simulink library "lib_rfsoc_fec"  (R2020b)
settings: Solver=VariableStepAuto  StartTime=0.0  StopTime=10.0  RelTol=1e-3
undefined symbols (not defined in the file): d, fs
libraries: hdlsllib x42, commseqgen3 x28, simulink x17, dspsigops x10
(part 1 of 2)
settings Model: Creator=ckb13136  LastModifiedBy=ckb13136

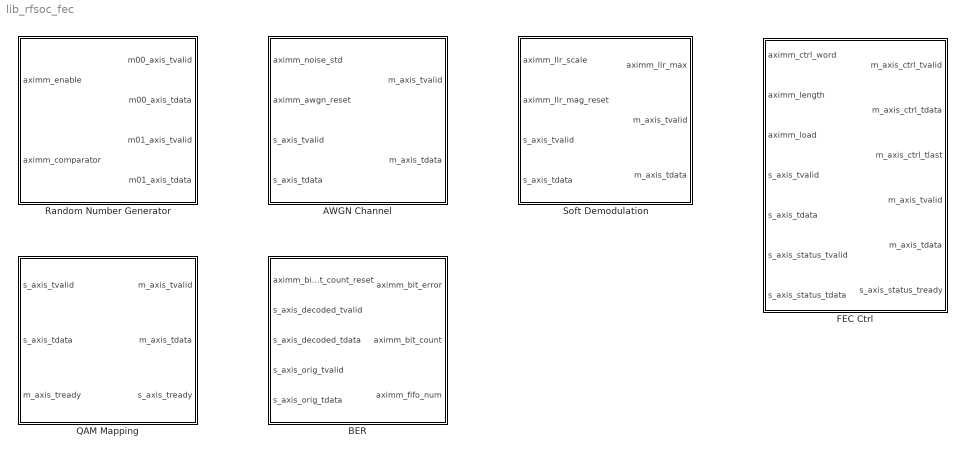
== system lib_rfsoc_fec ==
  AWGN Channel : Subsystem  TreatAsAtomicUnit=on
  BER : Subsystem  TreatAsAtomicUnit=on
  FEC Ctrl : Subsystem  TreatAsAtomicUnit=on
  QAM Mapping : Subsystem  TreatAsAtomicUnit=on
  Random Number Generator : Subsystem  TreatAsAtomicUnit=on
  Soft Demodulation : Subsystem  TreatAsAtomicUnit=on

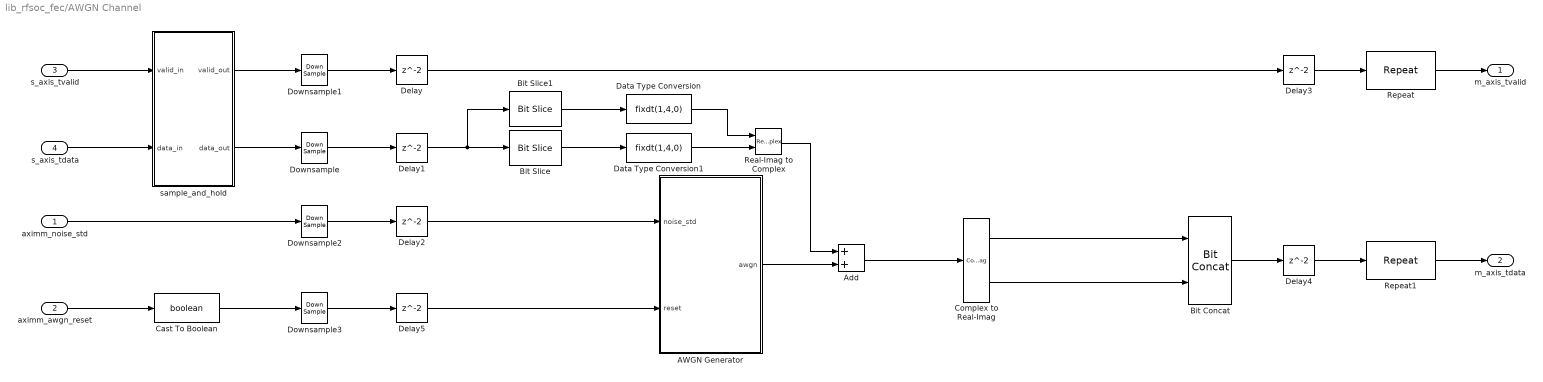
== system lib_rfsoc_fec/AWGN Channel ==
  aximm_noise_std : Inport
  aximm_awgn_reset : Inport  Port=2
  s_axis_tvalid : Inport  Port=3
  s_axis_tdata : Inport  Port=4
  AWGN Generator : Subsystem
  Add : Sum  OutDataTypeStr=fixdt(1,16,11)  SaturateOnIntegerOverflow=on
  Bit Concat : hdlsllib/Logic and Bit Operations/Bit Concat  numInputs=2
  Bit Slice : hdlsllib/Logic and Bit Operations/Bit Slice  lidx=3  ridx=0
      settings: SourceProductBaseCode=SL
  Bit Slice1 : hdlsllib/Logic and Bit Operations/Bit Slice  lidx=7  ridx=4
      settings: SourceProductBaseCode=SL
  Cast To Boolean : DataTypeConversion  OutDataTypeStr=boolean
  Complex to Real-Imag : ComplexToRealImag
  Data Type Conversion : DataTypeConversion  OutDataTypeStr=fixdt(1,4,0)  ConvertRealWorld=Stored Integer (SI)
  Data Type Conversion1 : DataTypeConversion  OutDataTypeStr=fixdt(1,4,0)  ConvertRealWorld=Stored Integer (SI)
  Delay{,1..5} (6 alike) : Delay
  Downsample{,1..3} (4 alike) : DownSample  N=4  RateOptions=Allow multirate processing
  Real-Imag to Complex : RealImagToComplex
  Repeat : dspsigops/Repeat  N=4  InputProcessing=Columns as channels (frame based)  RateOptions=Allow multirate processing  ic=0  mode=Unused parameter value
      settings: SourceProductName=DSP System Toolbox
  Repeat1 : dspsigops/Repeat  N=4  InputProcessing=Columns as channels (frame based)  RateOptions=Allow multirate processing  ic=0  mode=Unused parameter value
      settings: SourceProductName=DSP System Toolbox
  sample_and_hold : Subsystem
  m_axis_tvalid : Outport
  m_axis_tdata : Outport  Port=2
  wires:
  AWGN Generator/1(awgn) -> Add/2
  aximm_noise_std/1 -> Downsample2/1
  Delay2/1 -> AWGN Generator/1(noise_std)
  Downsample2/1 -> Delay2/1
  Delay5/1 -> AWGN Generator/2(reset)
  sample_and_hold/1(" valid_out") -> Downsample1/1
  Downsample1/1 -> Delay/1
  Downsample/1 -> Delay1/1
  Delay/1 -> Delay3/1
  sample_and_hold/2(" data_out") -> Downsample/1
  s_axis_tvalid/1 -> sample_and_hold/1(valid_in)
  s_axis_tdata/1 -> sample_and_hold/2(data_in)
  Delay1/1 -> Bit Slice1/1, Bit Slice/1
  Repeat1/1 -> m_axis_tdata/1
  Repeat/1 -> m_axis_tvalid/1
  Delay3/1 -> Repeat/1
  Delay4/1 -> Repeat1/1
  Bit Slice1/1 -> Data Type Conversion/1
  Bit Slice/1 -> Data Type Conversion1/1
  Data Type Conversion/1 -> Real-Imag to Complex/1
  Data Type Conversion1/1 -> Real-Imag to Complex/2
  Real-Imag to Complex/1 -> Add/1
  Add/1 -> Complex to Real-Imag/1
  Bit Concat/1 -> Delay4/1
  Complex to Real-Imag/1 -> Bit Concat/1
  Complex to Real-Imag/2 -> Bit Concat/2
  Downsample3/1 -> Delay5/1
  aximm_awgn_reset/1 -> Cast To Boolean/1
  Cast To Boolean/1 -> Downsample3/1

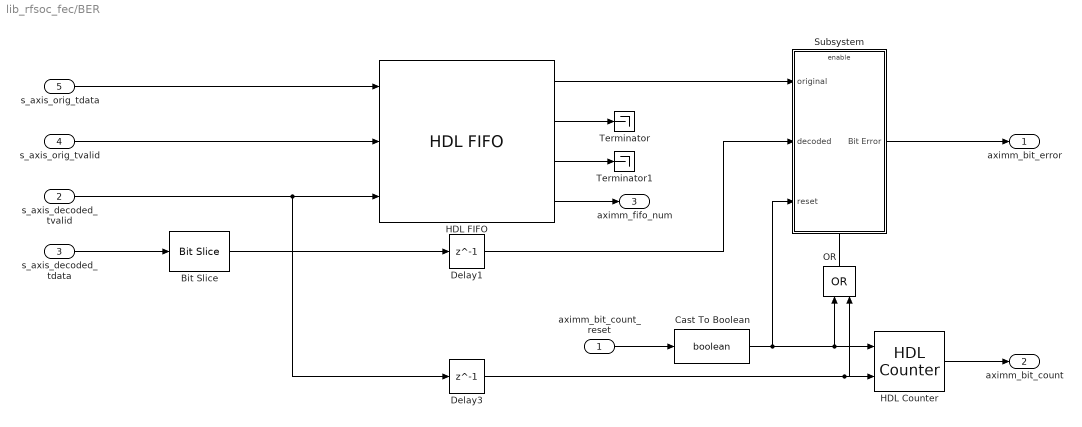
== system lib_rfsoc_fec/BER ==
  aximm_bit_count_reset : Inport
  s_axis_decoded_tvalid : Inport  Port=2
  s_axis_decoded_tdata : Inport  Port=3
  s_axis_orig_tvalid : Inport  Port=4
  s_axis_orig_tdata : Inport  Port=5
  Bit Slice : hdlsllib/Logic and Bit Operations/Bit Slice  lidx=7  ridx=0
      settings: SourceProductBaseCode=SL
  Cast To Boolean : DataTypeConversion  OutDataTypeStr=boolean
  Delay1 : Delay  DelayLength=1
  Delay3 : Delay  DelayLength=1
  HDL Counter : hdlsllib/Sources/HDL Counter  CountType=Free running  CountInit=0  CountStep=8  CountMax=25  CountFromType=Initial value  CountFrom=0  CountResetPort=on  CountLoadPort=off  CountEnbPort=on  CountDirPort=off  CountDataType=Unsigned  CountWordLen=32  CountFracLen=0  CountSampTime=1
  HDL FIFO : hdlsllib/HDL RAMs/HDL FIFO  fifo_size=8192  mode=Classic  ratio=1  push_msg=Warning  pop_msg=Warning  show_empty=on  show_full=on  show_num=on  LabelModeActiveChoice_Mode=Classic
      settings: SourceProductBaseCode=SL
  OR : Logic  Operator=OR  IconShape=distinctive  AllPortsSameDT=off  OutDataTypeStr=boolean
  Subsystem : Subsystem
  Terminator : Terminator
  Terminator1 : Terminator
  aximm_bit_error : Outport
  aximm_bit_count : Outport  Port=2
  aximm_fifo_num : Outport  Port=3
  wires:
  HDL FIFO/4 -> aximm_fifo_num/1
  HDL FIFO/2 -> Terminator/1
  s_axis_decoded_tvalid/1 -> HDL FIFO/3, Delay3/1
  Delay3/1 -> OR/2, HDL Counter/2
  s_axis_decoded_tdata/1 -> Bit Slice/1
  s_axis_orig_tvalid/1 -> HDL FIFO/2
  HDL FIFO/3 -> Terminator1/1
  Subsystem/1(Bit Error) -> aximm_bit_error/1
  HDL FIFO/1 -> Subsystem/1(original)
  Delay1/1 -> Subsystem/2(decoded)
  HDL Counter/1 -> aximm_bit_count/1
  Bit Slice/1 -> Delay1/1
  s_axis_orig_tdata/1 -> HDL FIFO/1
  aximm_bit_count_reset/1 -> Cast To Boolean/1
  Cast To Boolean/1 -> OR/1, HDL Counter/1, Subsystem/3(reset)
  OR/1 -> Subsystem/Enable

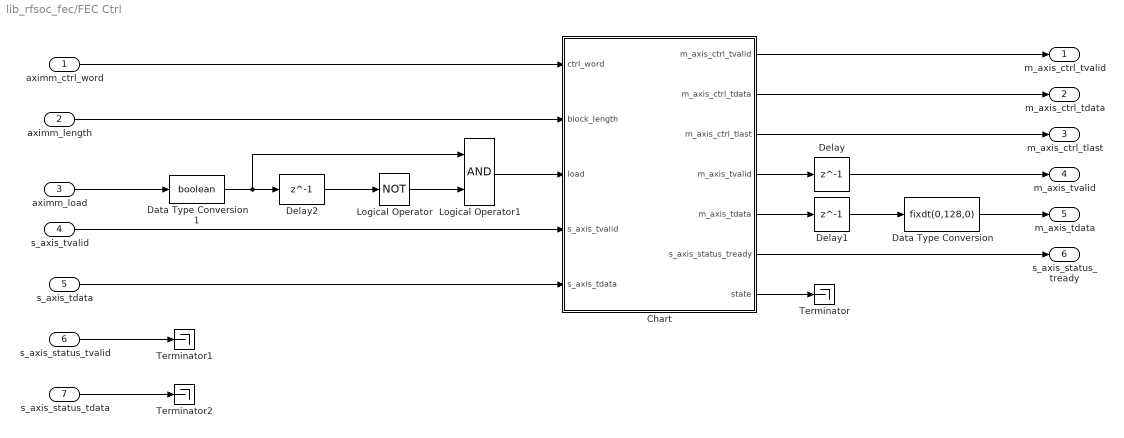
== system lib_rfsoc_fec/FEC Ctrl ==
  aximm_ctrl_word : Inport
  aximm_length : Inport  Port=2
  aximm_load : Inport  Port=3
  s_axis_tvalid : Inport  Port=4
  s_axis_tdata : Inport  Port=5
  s_axis_status_tvalid : Inport  Port=6
  s_axis_status_tdata : Inport  Port=7
  Chart : Stateflow chart  TreatAsAtomicUnit=on
  Data Type Conversion : DataTypeConversion  OutDataTypeStr=fixdt(0,128,0)
  Data Type Conversion1 : DataTypeConversion  OutDataTypeStr=boolean  SaturateOnIntegerOverflow=on  RndMeth=Zero
  Delay : Delay  DelayLength=1
  Delay1 : Delay  DelayLength=1
  Delay2 : Delay  DelayLength=1  InitialCondition=1  InputProcessing=Columns as channels (frame based)
  Logical Operator : Logic  Operator=NOT  Inputs=1
  Logical Operator1 : Logic
  Terminator : Terminator
  Terminator1 : Terminator
  Terminator2 : Terminator
  m_axis_ctrl_tvalid : Outport
  m_axis_ctrl_tdata : Outport  Port=2
  m_axis_ctrl_tlast : Outport  Port=3
  m_axis_tvalid : Outport  Port=4
  m_axis_tdata : Outport  Port=5
  s_axis_status_tready : Outport  Port=6
  wires:
  Chart/3(m_axis_ctrl_tlast) -> m_axis_ctrl_tlast/1
  Chart/7(state) -> Terminator/1
  aximm_length/1 -> Chart/2(block_length)
  s_axis_tvalid/1 -> Chart/4(s_axis_tvalid)
  s_axis_tdata/1 -> Chart/5(s_axis_tdata)
  aximm_ctrl_word/1 -> Chart/1(ctrl_word)
  Chart/2(m_axis_ctrl_tdata) -> m_axis_ctrl_tdata/1
  Chart/4(m_axis_tvalid) -> Delay/1
  Chart/5(m_axis_tdata) -> Delay1/1
  Chart/6(s_axis_status_tready) -> s_axis_status_tready/1
  Chart/1(m_axis_ctrl_tvalid) -> m_axis_ctrl_tvalid/1
  Delay/1 -> m_axis_tvalid/1
  Delay1/1 -> Data Type Conversion/1
  Data Type Conversion/1 -> m_axis_tdata/1
  Logical Operator1/1 -> Chart/3(load)
  s_axis_status_tvalid/1 -> Terminator1/1
  s_axis_status_tdata/1 -> Terminator2/1
  Logical Operator/1 -> Logical Operator1/2
  Data Type Conversion1/1 -> Delay2/1, Logical Operator1/1
  Delay2/1 -> Logical Operator/1
  aximm_load/1 -> Data Type Conversion1/1

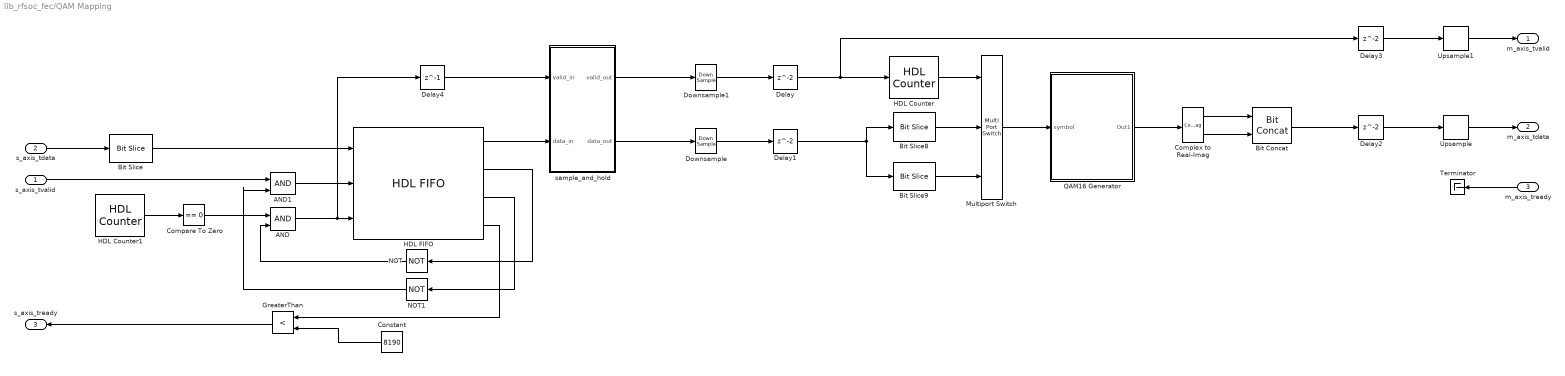
== system lib_rfsoc_fec/QAM Mapping ==
  s_axis_tvalid : Inport
  s_axis_tdata : Inport  Port=2
  m_axis_tready : Inport  Port=3
  AND : Logic  IconShape=distinctive  AllPortsSameDT=off  OutDataTypeStr=boolean
  AND1 : Logic  IconShape=distinctive  AllPortsSameDT=off  OutDataTypeStr=boolean
  Bit Concat : hdlsllib/Logic and Bit Operations/Bit Concat  numInputs=2
  Bit Slice : hdlsllib/Logic and Bit Operations/Bit Slice  lidx=7  ridx=0
      settings: SourceProductBaseCode=SL
  Bit Slice8 : hdlsllib/Logic and Bit Operations/Bit Slice  lidx=3  ridx=0
      settings: SourceProductBaseCode=SL
  Bit Slice9 : hdlsllib/Logic and Bit Operations/Bit Slice  lidx=7  ridx=4
      settings: SourceProductBaseCode=SL
  Compare To Zero : simulink/Logic and Bit Operations/Compare To Zero  relop===  OutDataTypeStr=boolean
  Complex to Real-Imag : ComplexToRealImag
  Constant : Constant  Value=8190  OutDataTypeStr=fixdt(0,log2(8190),0)  SampleTime=1/(fs*16)
  Delay{,1..3} (4 alike) : Delay
  Delay4 : Delay  DelayLength=1
  Downsample : DownSample  N=4  RateOptions=Allow multirate processing
  Downsample1 : DownSample  N=4  RateOptions=Allow multirate processing
  GreaterThan : RelationalOperator  Operator=<  OutDataTypeStr=boolean  RndMeth=Simplest
  HDL Counter : hdlsllib/Sources/HDL Counter  CountType=Count limited  CountInit=0  CountStep=1  CountMax=1  CountFromType=Initial value  CountFrom=0  CountResetPort=off  CountLoadPort=off  CountEnbPort=on  CountDirPort=off  CountDataType=Unsigned  CountWordLen=1  CountFracLen=0  CountSampTime=1/(fs*2)
  HDL Counter1 : hdlsllib/Sources/HDL Counter  CountType=Free running  CountInit=0  CountStep=1  CountMax=1  CountFromType=Initial value  CountFrom=0  CountResetPort=off  CountLoadPort=off  CountEnbPort=off  CountDirPort=off  CountDataType=Unsigned  CountWordLen=3  CountFracLen=0  CountSampTime=1/(fs*16)
  HDL FIFO : hdlsllib/HDL RAMs/HDL FIFO  fifo_size=8192  mode=Classic  ratio=1  push_msg=Warning  pop_msg=Warning  show_empty=on  show_full=on  show_num=on  LabelModeActiveChoice_Mode=Classic
      settings: SourceProductBaseCode=SL
  Multiport Switch : MultiPortSwitch  DataPortOrder=Zero-based contiguous  Inputs=2  zeroidx=on
  NOT : Logic  Operator=NOT  IconShape=distinctive  AllPortsSameDT=off  OutDataTypeStr=boolean
  NOT1 : Logic  Operator=NOT  IconShape=distinctive  AllPortsSameDT=off  OutDataTypeStr=boolean
  QAM16 Generator : Subsystem
  Terminator : Terminator
  Upsample : dspsigops/Upsample  N=4  phase=0  RateOptions=Allow multirate processing  ic=0  mode=Unused parameter value
  Upsample1 : dspsigops/Upsample  N=4  phase=0  RateOptions=Allow multirate processing  ic=0  mode=Unused parameter value
  sample_and_hold : Subsystem
  m_axis_tvalid : Outport
  m_axis_tdata : Outport  Port=2
  s_axis_tready : Outport  Port=3
  wires:
  Bit Slice9/1 -> Multiport Switch/3
  Bit Slice8/1 -> Multiport Switch/2
  HDL Counter/1 -> Multiport Switch/1
  Multiport Switch/1 -> QAM16 Generator/1(symbol)
  Downsample/1 -> Delay1/1
  sample_and_hold/1(" valid_out") -> Downsample1/1
  sample_and_hold/2(" data_out") -> Downsample/1
  Downsample1/1 -> Delay/1
  HDL FIFO/1 -> sample_and_hold/2(data_in)
  Delay/1 -> Delay3/1, HDL Counter/1
  Delay1/1 -> Bit Slice9/1, Bit Slice8/1
  Delay2/1 -> Upsample/1
  Delay3/1 -> Upsample1/1
  Upsample1/1 -> m_axis_tvalid/1
  Upsample/1 -> m_axis_tdata/1
  QAM16 Generator/1(Out1) -> Complex to Real-Imag/1
  Complex to Real-Imag/1 -> Bit Concat/1
  Complex to Real-Imag/2 -> Bit Concat/2
  Bit Concat/1 -> Delay2/1
  m_axis_tready/1 -> Terminator/1
  s_axis_tvalid/1 -> AND1/1
  s_axis_tdata/1 -> Bit Slice/1
  Bit Slice/1 -> HDL FIFO/1
  HDL FIFO/2 -> NOT/1
  AND/1 -> Delay4/1, HDL FIFO/3
  NOT/1 -> AND/2
  Constant/1 -> GreaterThan/2
  AND1/1 -> HDL FIFO/2
  HDL FIFO/3 -> NOT1/1
  NOT1/1 -> AND1/2
  HDL FIFO/4 -> GreaterThan/1
  GreaterThan/1 -> s_axis_tready/1
  HDL Counter1/1 -> Compare To Zero/1
  Compare To Zero/1 -> AND/1
  Delay4/1 -> sample_and_hold/1(valid_in)

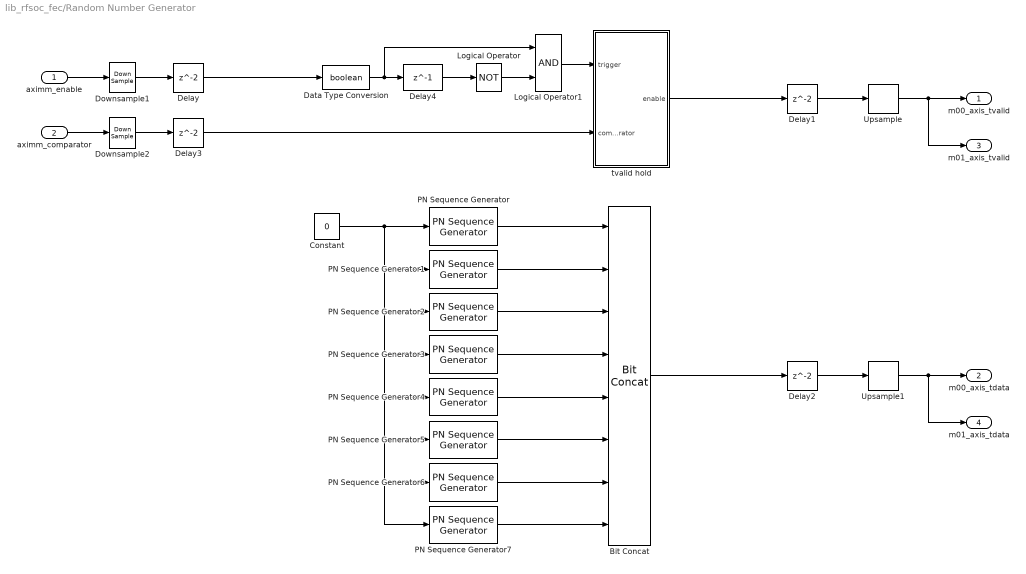
== system lib_rfsoc_fec/Random Number Generator ==
  aximm_enable : Inport
  aximm_comparator : Inport  Port=2
  Bit Concat : hdlsllib/Logic and Bit Operations/Bit Concat  numInputs=8
  Constant : Constant  Value=0  OutDataTypeStr=boolean  SampleTime=1/fs
  Data Type Conversion : DataTypeConversion  OutDataTypeStr=boolean  SaturateOnIntegerOverflow=on  RndMeth=Zero
  Delay{,1..3} (4 alike) : Delay
  Delay4 : Delay  DelayLength=1  InitialCondition=1  InputProcessing=Columns as channels (frame based)
  Downsample1 : DownSample  N=16  RateOptions=Allow multirate processing
  Downsample2 : DownSample  N=16  RateOptions=Allow multirate processing
  Logical Operator : Logic  Operator=NOT  Inputs=1
  Logical Operator1 : Logic
  PN Sequence Generator : commseqgen3/PN Sequence Generator  poly='z^13 + z^12 + z^11 + z^8 + 1'  ini_sta=[0 1 1 0 0 0 0 0 0 1 0 0 0]  outBitMaskSource=Dialog parameter  shift=0  outVarSiz=off  maxOutSizeMode=Dialog parameter  maxOutSize=[10 1]  Ts=-1  sampPerFrame=1  reset=on  bitPackedOutputs=off  outDataType=boolean  numPackedBits=8  bitPackDataSigned=off  bitPackedOutDType=Smallest integer
  PN Sequence Generator1 : commseqgen3/PN Sequence Generator  poly='z^13 + z^12 + z^11 + z^8 + 1'  ini_sta=[0 0 1 1 0 0 0 0 0 0 0 1 1]  outBitMaskSource=Dialog parameter  shift=0  outVarSiz=off  maxOutSizeMode=Dialog parameter  maxOutSize=[10 1]  Ts=-1  sampPerFrame=1  reset=on  bitPackedOutputs=off  outDataType=boolean  numPackedBits=8  bitPackDataSigned=off  bitPackedOutDType=Smallest integer
  PN Sequence Generator2 : commseqgen3/PN Sequence Generator  poly='z^13 + z^12 + z^11 + z^8 + 1'  ini_sta=[1 1 0 1 0 0 0 0 0 1 0 0 1]  outBitMaskSource=Dialog parameter  shift=0  outVarSiz=off  maxOutSizeMode=Dialog parameter  maxOutSize=[10 1]  Ts=-1  sampPerFrame=1  reset=on  bitPackedOutputs=off  outDataType=boolean  numPackedBits=8  bitPackDataSigned=off  bitPackedOutDType=Smallest integer
  PN Sequence Generator3 : commseqgen3/PN Sequence Generator  poly='z^13 + z^12 + z^11 + z^8 + 1'  ini_sta=[1 0 1 0 0 0 0 1 0 0 1 1 0]  outBitMaskSource=Dialog parameter  shift=0  outVarSiz=off  maxOutSizeMode=Dialog parameter  maxOutSize=[10 1]  Ts=-1  sampPerFrame=1  reset=on  bitPackedOutputs=off  outDataType=boolean  numPackedBits=8  bitPackDataSigned=off  bitPackedOutDType=Smallest integer
  PN Sequence Generator4 : commseqgen3/PN Sequence Generator  poly='z^13 + z^12 + z^11 + z^8 + 1'  ini_sta=[0 0 0 0 1 0 0 0 0 1 1 1 0]  outBitMaskSource=Dialog parameter  shift=0  outVarSiz=off  maxOutSizeMode=Dialog parameter  maxOutSize=[10 1]  Ts=-1  sampPerFrame=1  reset=on  bitPackedOutputs=off  outDataType=boolean  numPackedBits=8  bitPackDataSigned=off  bitPackedOutDType=Smallest integer
  PN Sequence Generator5 : commseqgen3/PN Sequence Generator  poly='z^13 + z^12 + z^11 + z^8 + 1'  ini_sta=[1 1 0 0 1 1 0 0 1 0 1 0 0]  outBitMaskSource=Dialog parameter  shift=0  outVarSiz=off  maxOutSizeMode=Dialog parameter  maxOutSize=[10 1]  Ts=-1  sampPerFrame=1  reset=on  bitPackedOutputs=off  outDataType=boolean  numPackedBits=8  bitPackDataSigned=off  bitPackedOutDType=Smallest integer
  PN Sequence Generator6 : commseqgen3/PN Sequence Generator  poly='z^13 + z^12 + z^11 + z^8 + 1'  ini_sta=[1 0 0 0 0 1 0 0 0 0 1 1 1]  outBitMaskSource=Dialog parameter  shift=0  outVarSiz=off  maxOutSizeMode=Dialog parameter  maxOutSize=[10 1]  Ts=-1  sampPerFrame=1  reset=on  bitPackedOutputs=off  outDataType=boolean  numPackedBits=8  bitPackDataSigned=off  bitPackedOutDType=Smallest integer
  PN Sequence Generator7 : commseqgen3/PN Sequence Generator  poly='z^13 + z^12 + z^11 + z^8 + 1'  ini_sta=[1 0 0 1 1 1 1 1 0 0 0 1 1]  outBitMaskSource=Dialog parameter  shift=0  outVarSiz=off  maxOutSizeMode=Dialog parameter  maxOutSize=[10 1]  Ts=-1  sampPerFrame=1  reset=on  bitPackedOutputs=off  outDataType=boolean  numPackedBits=8  bitPackDataSigned=off  bitPackedOutDType=Smallest integer
  Upsample : dspsigops/Upsample  N=16  phase=0  RateOptions=Allow multirate processing  ic=0  mode=Unused parameter value
  Upsample1 : dspsigops/Upsample  N=16  phase=0  RateOptions=Allow multirate processing  ic=0  mode=Unused parameter value
  tvalid hold : Subsystem
  m00_axis_tvalid : Outport
  m00_axis_tdata : Outport  Port=2
  m01_axis_tvalid : Outport  Port=3
  m01_axis_tdata : Outport  Port=4
  wires:
  Constant/1 -> PN Sequence Generator7/1, PN Sequence Generator6/1, PN Sequence Generator5/1, PN Sequence Generator4/1, PN Sequence Generator3/1, PN Sequence Generator2/1, PN Sequence Generator1/1, PN Sequence Generator/1
  PN Sequence Generator4/1 -> Bit Concat/5
  PN Sequence Generator7/1 -> Bit Concat/8
  PN Sequence Generator5/1 -> Bit Concat/6
  PN Sequence Generator/1 -> Bit Concat/1
  PN Sequence Generator3/1 -> Bit Concat/4
  PN Sequence Generator1/1 -> Bit Concat/2
  PN Sequence Generator2/1 -> Bit Concat/3
  PN Sequence Generator6/1 -> Bit Concat/7
  Bit Concat/1 -> Delay2/1
  tvalid hold/1(enable) -> Delay1/1
  aximm_enable/1 -> Downsample1/1
  Upsample/1 -> m01_axis_tvalid/1, m00_axis_tvalid/1
  Upsample1/1 -> m01_axis_tdata/1, m00_axis_tdata/1
  Delay1/1 -> Upsample/1
  Delay2/1 -> Upsample1/1
  Downsample1/1 -> Delay/1
  Logical Operator1/1 -> tvalid hold/1(trigger)
  aximm_comparator/1 -> Downsample2/1
  Downsample2/1 -> Delay3/1
  Delay3/1 -> tvalid hold/2(comparator)
  Logical Operator/1 -> Logical Operator1/2
  Data Type Conversion/1 -> Delay4/1, Logical Operator1/1
  Delay4/1 -> Logical Operator/1
  Delay/1 -> Data Type Conversion/1

== system lib_rfsoc_fec/Soft Demodulation ==
  aximm_llr_scale : Inport
  aximm_llr_mag_reset : Inport  Port=2
  s_axis_tvalid : Inport  Port=3
  s_axis_tdata : Inport  Port=4
  Bit Slice : hdlsllib/Logic and Bit Operations/Bit Slice  lidx=15  ridx=0
      settings: SourceProductBaseCode=SL
  Bit Slice1 : hdlsllib/Logic and Bit Operations/Bit Slice  lidx=31  ridx=16
      settings: SourceProductBaseCode=SL
  Cast To Boolean : DataTypeConversion  OutDataTypeStr=boolean
  Data Type Conversion : DataTypeConversion  OutDataTypeStr=fixdt(1,16,11)  ConvertRealWorld=Stored Integer (SI)
  Data Type Conversion1 : DataTypeConversion  OutDataTypeStr=fixdt(1,16,11)  ConvertRealWorld=Stored Integer (SI)
  MATLAB Function : MATLAB Function  TreatAsAtomicUnit=on
  Soft Demodulation : Subsystem
  sign_extend : Subsystem
  symmetric_saturation : MATLAB Function  TreatAsAtomicUnit=on
  aximm_llr_max : Outport
  m_axis_tvalid : Outport  Port=2
  m_axis_tdata : Outport  Port=3
  wires:
  aximm_llr_scale/1 -> Soft Demodulation/4(LLR Scale)
  Soft Demodulation/1(LLR Values) -> symmetric_saturation/1(u), MATLAB Function/1(u)
  s_axis_tvalid/1 -> m_axis_tvalid/1, Soft Demodulation/1(valid)
  MATLAB Function/1(y) -> aximm_llr_max/1
  aximm_llr_mag_reset/1 -> Cast To Boolean/1
  sign_extend/1(y) -> m_axis_tdata/1
  symmetric_saturation/1(y) -> sign_extend/1(u)
  Cast To Boolean/1 -> MATLAB Function/2(reset)
  Bit Slice1/1 -> Data Type Conversion/1
  Bit Slice/1 -> Data Type Conversion1/1
  Data Type Conversion/1 -> Soft Demodulation/2(real)
  s_axis_tdata/1 -> Bit Slice1/1, Bit Slice/1
  Data Type Conversion1/1 -> Soft Demodulation/3(imag)

== system lib_rfsoc_fec/AWGN Channel/AWGN Generator ==
  noise_std : Inport
  reset : Inport  Port=2
  1-D Lookup Table : Lookup_n-D  NumberOfTableDimensions=1  BreakpointsForDimension1=[0:4095]  BreakpointsForDimension1DataTypeStr=fixdt(0,12,0)  IndexSearchMethod=Evenly spaced points  Table=d  InterpMethod=Flat  ExtrapMethod=Clip  DiagnosticForOutOfRangeInput=Error  InternalRulePriority=Speed  OutDataTypeStr=fixdt(1,18,14)  RndMeth=Simplest  InputSameDT=on
  Cosine Lookup : Lookup_n-D  NumberOfTableDimensions=1  BreakpointsForDimension1=[0:255]  IndexSearchMethod=Evenly spaced points  Table=cos([0:255]*2*pi/256)  InterpMethod=Flat  ExtrapMethod=Clip  DiagnosticForOutOfRangeInput=Error  UseLastTableValue=on  OutDataTypeStr=fixdt(1,16,14)  RndMeth=Simplest  InputSameDT=on
  Data Type Conversion : DataTypeConversion  OutDataTypeStr=fixdt(0,16,14)  RndMeth=Round  SaturateOnIntegerOverflow=on
  Gain : Gain  Gain=0.7  OutDataTypeStr=fixdt(1,15,11)  RndMeth=Nearest  SaturateOnIntegerOverflow=on
  Product : Product  OutDataTypeStr=fixdt(1,17,14)  RndMeth=Round  SaturateOnIntegerOverflow=on
  Product1 : Product  OutDataTypeStr=fixdt(1,17,14)  RndMeth=Round  SaturateOnIntegerOverflow=on
  Product3 : Product  OutDataTypeStr=fixdt(1,18,14)  RndMeth=Round
  Real-Imag to Complex1 : RealImagToComplex
  Sine Lookup : Lookup_n-D  NumberOfTableDimensions=1  BreakpointsForDimension1=[0:255]  IndexSearchMethod=Evenly spaced points  Table=sin([0:255]*2*pi/256)  InterpMethod=Flat  ExtrapMethod=Clip  DiagnosticForOutOfRangeInput=Error  UseLastTableValue=on  OutDataTypeStr=fixdt(1,16,14)  RndMeth=Simplest  InputSameDT=on
  Subsystem3 : Subsystem
  awgn : Outport
  wires:
  noise_std/1 -> Data Type Conversion/1
  Product1/1 -> Real-Imag to Complex1/1
  Product/1 -> Real-Imag to Complex1/2
  Product3/1 -> Gain/1
  Sine Lookup/1 -> Product/1
  reset/1 -> Subsystem3/1(Reset)
  Subsystem3/2(LFSR_F) -> 1-D Lookup Table/1
  1-D Lookup Table/1 -> Product1/2, Product/2
  Subsystem3/1(LFSR_G) -> Cosine Lookup/1, Sine Lookup/1
  Cosine Lookup/1 -> Product1/1
  Gain/1 -> awgn/1
  Real-Imag to Complex1/1 -> Product3/2
  Data Type Conversion/1 -> Product3/1

== system lib_rfsoc_fec/AWGN Channel/sample_and_hold ==
  valid_in : Inport
  data_in : Inport  Port=2
  Sample and Hold : dspsigops/Sample and Hold  trig=Rising edge  initCond=0  latchinput=off
  tvalid hold : Subsystem
  " valid_out" : Outport
  " data_out" : Outport  Port=2
  wires:
  valid_in/1 -> tvalid hold/1(In1), Sample and Hold/Trigger
  tvalid hold/1(" ") -> " valid_out"/1
  data_in/1 -> Sample and Hold/1
  Sample and Hold/1 -> " data_out"/1

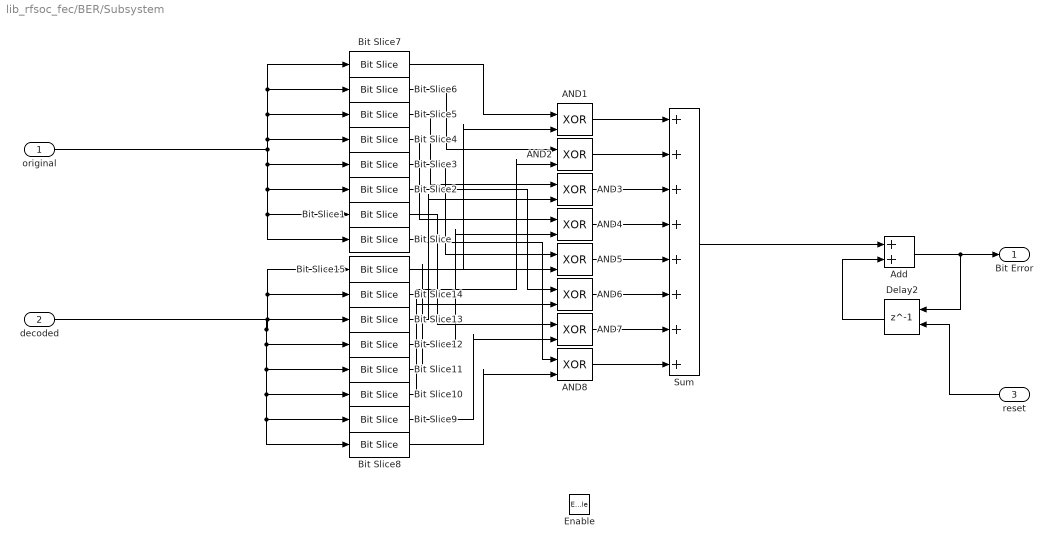
== system lib_rfsoc_fec/BER/Subsystem ==
  original : Inport
  decoded : Inport  Port=2
  reset : Inport  Port=3
  Enable : EnablePort
  AND{1..8} (8 alike) : Logic  Operator=XOR  IconShape=distinctive  AllPortsSameDT=off  OutDataTypeStr=boolean
  Add : Sum  OutDataTypeStr=uint32
  Bit Slice : hdlsllib/Logic and Bit Operations/Bit Slice  lidx=0  ridx=0
      settings: SourceProductBaseCode=SL
  Bit Slice1 : hdlsllib/Logic and Bit Operations/Bit Slice  lidx=1  ridx=1
      settings: SourceProductBaseCode=SL
  Bit Slice10 : hdlsllib/Logic and Bit Operations/Bit Slice  lidx=2  ridx=2
      settings: SourceProductBaseCode=SL
  Bit Slice11 : hdlsllib/Logic and Bit Operations/Bit Slice  lidx=3  ridx=3
      settings: SourceProductBaseCode=SL
  Bit Slice12 : hdlsllib/Logic and Bit Operations/Bit Slice  lidx=4  ridx=4
      settings: SourceProductBaseCode=SL
  Bit Slice13 : hdlsllib/Logic and Bit Operations/Bit Slice  lidx=5  ridx=5
      settings: SourceProductBaseCode=SL
  Bit Slice14 : hdlsllib/Logic and Bit Operations/Bit Slice  lidx=6  ridx=6
      settings: SourceProductBaseCode=SL
  Bit Slice15 : hdlsllib/Logic and Bit Operations/Bit Slice  lidx=7  ridx=7
      settings: SourceProductBaseCode=SL
  Bit Slice2 : hdlsllib/Logic and Bit Operations/Bit Slice  lidx=2  ridx=2
      settings: SourceProductBaseCode=SL
  Bit Slice3 : hdlsllib/Logic and Bit Operations/Bit Slice  lidx=3  ridx=3
      settings: SourceProductBaseCode=SL
  Bit Slice4 : hdlsllib/Logic and Bit Operations/Bit Slice  lidx=4  ridx=4
      settings: SourceProductBaseCode=SL
  Bit Slice5 : hdlsllib/Logic and Bit Operations/Bit Slice  lidx=5  ridx=5
      settings: SourceProductBaseCode=SL
  Bit Slice6 : hdlsllib/Logic and Bit Operations/Bit Slice  lidx=6  ridx=6
      settings: SourceProductBaseCode=SL
  Bit Slice7 : hdlsllib/Logic and Bit Operations/Bit Slice  lidx=7  ridx=7
      settings: SourceProductBaseCode=SL
  Bit Slice8 : hdlsllib/Logic and Bit Operations/Bit Slice  lidx=0  ridx=0
      settings: SourceProductBaseCode=SL
  Bit Slice9 : hdlsllib/Logic and Bit Operations/Bit Slice  lidx=1  ridx=1
      settings: SourceProductBaseCode=SL
  Delay2 : Delay  DelayLength=1  ExternalReset=Level
      settings: InputPortMap=u0,r5
  Sum : Sum  Inputs=++++++++  OutDataTypeStr=fixdt(0,3,0)  SaturateOnIntegerOverflow=on
  Bit Error : Outport  InitialOutput=0
  wires:
  Bit Slice14/1 -> AND2/2
  original/1 -> Bit Slice/1, Bit Slice1/1, Bit Slice2/1, Bit Slice3/1, Bit Slice4/1, Bit Slice5/1, Bit Slice6/1, Bit Slice7/1
  AND5/1 -> Sum/5
  Delay2/1 -> Add/2
  Bit Slice15/1 -> AND1/2
  AND2/1 -> Sum/2
  Bit Slice6/1 -> AND2/1
  AND4/1 -> Sum/4
  decoded/1 -> Bit Slice8/1, Bit Slice9/1, Bit Slice10/1, Bit Slice11/1, Bit Slice12/1, Bit Slice13/1, Bit Slice15/1, Bit Slice14/1
  AND6/1 -> Sum/6
  Sum/1 -> Add/1
  AND7/1 -> Sum/7
  Bit Slice2/1 -> AND6/1
  AND8/1 -> Sum/8
  Bit Slice/1 -> AND8/1
  Bit Slice4/1 -> AND4/1
  Bit Slice3/1 -> AND5/1
  Bit Slice5/1 -> AND3/1
  Bit Slice7/1 -> AND1/1
  Bit Slice8/1 -> AND8/2
  Add/1 -> Bit Error/1, Delay2/1
  Bit Slice10/1 -> AND6/2
  Bit Slice12/1 -> AND4/2
  Bit Slice9/1 -> AND7/2
  Bit Slice1/1 -> AND7/1
  AND3/1 -> Sum/3
  Bit Slice13/1 -> AND3/2
  Bit Slice11/1 -> AND5/2
  AND1/1 -> Sum/1
  reset/1 -> Delay2/2

== system lib_rfsoc_fec/QAM Mapping/QAM16 Generator ==
  symbol : Inport
  Bit Slice1 : hdlsllib/Logic and Bit Operations/Bit Slice  lidx=1  ridx=0
      settings: SourceProductBaseCode=SL
  Bit Slice2 : hdlsllib/Logic and Bit Operations/Bit Slice  lidx=3  ridx=2
      settings: SourceProductBaseCode=SL
  Constant1 : Constant  Value=3  OutDataTypeStr=fixdt(1,3,0)  SampleTime=1/(4*fs)
  Constant2 : Constant  OutDataTypeStr=fixdt(1,3,0)  SampleTime=1/(4*fs)
  Constant3 : Constant  Value=-1  OutDataTypeStr=fixdt(1,3,0)  SampleTime=1/(4*fs)
  Constant4 : Constant  Value=-3  OutDataTypeStr=fixdt(1,3,0)  SampleTime=1/(4*fs)
  Data Type Conversion : DataTypeConversion  OutDataTypeStr=fixdt(1,4,0)
  Multiport Switch : MultiPortSwitch  DataPortOrder=Zero-based contiguous  Inputs=4  zeroidx=on
  Multiport Switch1 : MultiPortSwitch  DataPortOrder=Zero-based contiguous  Inputs=4  zeroidx=on
  Real-Imag to Complex : RealImagToComplex
  Out1 : Outport
  wires:
  Real-Imag to Complex/1 -> Data Type Conversion/1
  Bit Slice1/1 -> Multiport Switch1/1
  Multiport Switch1/1 -> Real-Imag to Complex/2
  Multiport Switch/1 -> Real-Imag to Complex/1
  Bit Slice2/1 -> Multiport Switch/1
  symbol/1 -> Bit Slice1/1, Bit Slice2/1
  Constant3/1 -> Multiport Switch/3, Multiport Switch1/5
  Constant4/1 -> Multiport Switch/2, Multiport Switch1/4
  Constant1/1 -> Multiport Switch/4, Multiport Switch1/2
  Constant2/1 -> Multiport Switch/5, Multiport Switch1/3
  Data Type Conversion/1 -> Out1/1

== system lib_rfsoc_fec/QAM Mapping/sample_and_hold ==
  valid_in : Inport
  data_in : Inport  Port=2
  Sample and Hold : dspsigops/Sample and Hold  trig=Rising edge  initCond=0  latchinput=off
  tvalid hold : Subsystem
  " valid_out" : Outport
  " data_out" : Outport  Port=2
  wires:
  valid_in/1 -> tvalid hold/1(In1), Sample and Hold/Trigger
  tvalid hold/1(" ") -> " valid_out"/1
  data_in/1 -> Sample and Hold/1
  Sample and Hold/1 -> " data_out"/1

== system lib_rfsoc_fec/Random Number Generator/tvalid hold ==
  trigger : Inport
  comparator : Inport  Port=2
  Delay2 : Delay  DelayLength=1
  Equal : RelationalOperator  Operator===  OutDataTypeStr=boolean  RndMeth=Simplest
  HDL Counter : hdlsllib/Sources/HDL Counter  CountType=Free running  CountInit=0  CountStep=1  CountMax=25  CountFromType=Initial value  CountFrom=0  CountResetPort=on  CountLoadPort=off  CountEnbPort=on  CountDirPort=off  CountDataType=Unsigned  CountWordLen=32  CountFracLen=0  CountSampTime=1
  Multiport Switch : MultiPortSwitch  DataPortOrder=Zero-based contiguous  Inputs=2  zeroidx=on
  OR : Logic  Operator=OR  IconShape=distinctive  AllPortsSameDT=off  OutDataTypeStr=boolean
  enable : Outport
  wires:
  HDL Counter/1 -> Equal/1
  Equal/1 -> HDL Counter/1, OR/1
  trigger/1 -> Multiport Switch/3, OR/2
  comparator/1 -> Equal/2
  Multiport Switch/1 -> HDL Counter/2, enable/1, Delay2/1
  Delay2/1 -> Multiport Switch/2
  OR/1 -> Multiport Switch/1

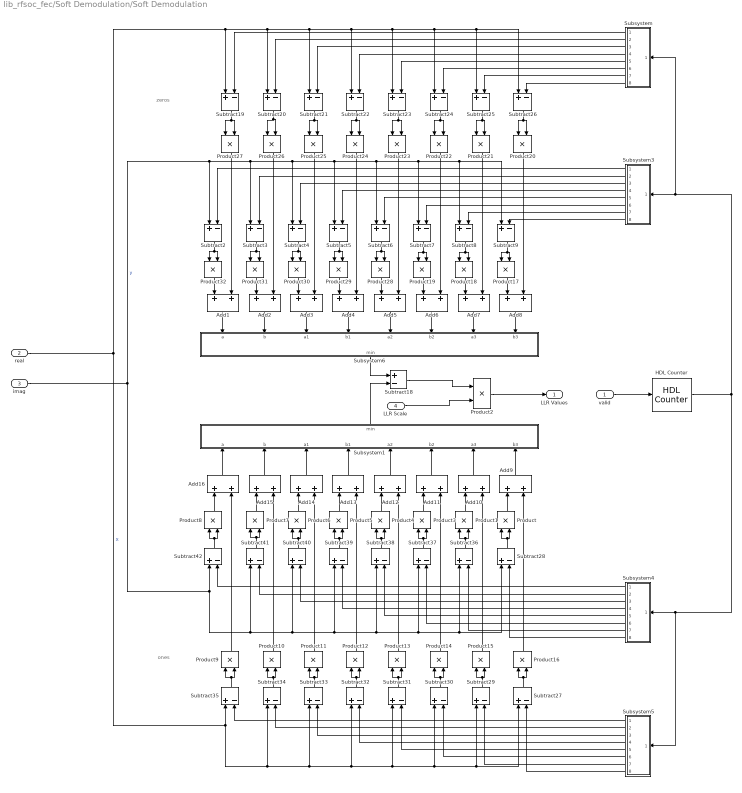
== system lib_rfsoc_fec/Soft Demodulation/Soft Demodulation ==
  note: ones
  note: zeros
  valid : Inport
  real : Inport  Port=2
  imag : Inport  Port=3
  LLR Scale : Inport  Port=4
  Add{1..16} (16 alike) : Sum  OutDataTypeStr=fixdt(1,35,22)  SaturateOnIntegerOverflow=on
  HDL Counter : hdlsllib/Sources/HDL Counter  CountType=Count limited  CountInit=0  CountStep=1  CountMax=3  CountFromType=Initial value  CountFrom=0  CountResetPort=off  CountLoadPort=off  CountEnbPort=on  CountDirPort=off  CountDataType=Unsigned  CountWordLen=2  CountFracLen=0  CountSampTime=1/(fs*2)
  Product{,1,3..16} (16 alike) : Product  SaturateOnIntegerOverflow=on
  Product{17..32} (16 alike) : Product
  Product2 : Product  OutDataTypeStr=fixdt(1,24,12)  RndMeth=Round  SaturateOnIntegerOverflow=on
  Subsystem : Subsystem
  Subsystem1 : Subsystem
  Subsystem3 : Subsystem
  Subsystem4 : Subsystem
  Subsystem5 : Subsystem
  Subsystem6 : Subsystem
  Subtract18 : Sum  Inputs=+-  OutDataTypeStr=fixdt(1,35,22)  SaturateOnIntegerOverflow=on
  Subtract{2..9,19..42} (32 alike) : Sum  Inputs=+-  OutDataTypeStr=fixdt(1,17,11)  SaturateOnIntegerOverflow=on
  LLR Values : Outport
  wires:
  HDL Counter/1 -> Subsystem3/1(enb), Subsystem/1(enb), Subsystem4/1(enb), Subsystem5/1(enb)
  valid/1 -> HDL Counter/1
  Subsystem/8(Out8) -> Subtract26/2
  Subsystem/7(Out7) -> Subtract25/2
  Subsystem/6(Out6) -> Subtract24/2
  Subsystem/5(Out5) -> Subtract23/2
  Subsystem/4(Out4) -> Subtract22/2
  Subsystem/3(Out3) -> Subtract21/2
  Subsystem/2(Out2) -> Subtract20/2
  Subsystem/1(Out1) -> Subtract19/2
  Subtract7/1 -> Product19/2, Product19/1
  Subtract22/1 -> Product24/2, Product24/1
  Subtract20/1 -> Product26/1, Product26/2
  Subtract8/1 -> Product18/2, Product18/1
  Subtract9/1 -> Product17/1, Product17/2
  Subtract27/1 -> Product16/2, Product16/1
  Subtract29/1 -> Product15/2, Product15/1
  Subtract30/1 -> Product14/2, Product14/1
  Subtract31/1 -> Product13/2, Product13/1
  Subtract32/1 -> Product12/2, Product12/1
  Subtract33/1 -> Product11/2, Product11/1
  Subtract37/1 -> Product3/2, Product3/1
  Product2/1 -> LLR Values/1
  Subsystem5/5(Out5) -> Subtract31/2
  Subtract28/1 -> Product/1, Product/2
  Add5/1 -> Subsystem6/5(a2)
  Subsystem3/8(Out8) -> Subtract9/2
  Add4/1 -> Subsystem6/4(b1)
  Product11/1 -> Add14/2
  Product29/1 -> Add4/1
  Subsystem4/8(Out8) -> Subtract28/2
  Subsystem4/2(Out2) -> Subtract41/2
  Subsystem5/8(Out8) -> Subtract27/2
  Subsystem5/7(Out7) -> Subtract29/2
  Subtract40/1 -> Product6/1, Product6/2
  Subtract34/1 -> Product10/1, Product10/2
  Product32/1 -> Add1/1
  Subsystem5/1(Out1) -> Subtract35/2
  Subtract39/1 -> Product5/1, Product5/2
  Subsystem3/7(Out7) -> Subtract8/2
  Product16/1 -> Add9/2
  Subsystem4/1(Out1) -> Subtract42/2
  Subsystem5/6(Out6) -> Subtract30/2
  Product24/1 -> Add4/2
  Subtract3/1 -> Product31/2, Product31/1
  Product13/1 -> Add12/2
  Subsystem5/3(Out3) -> Subtract33/2
  Subsystem5/2(Out2) -> Subtract34/2
  Subsystem4/3(Out3) -> Subtract40/2
  Product17/1 -> Add8/1
  Subsystem4/4(Out4) -> Subtract39/2
  Product9/1 -> Add16/2
  Add15/1 -> Subsystem1/2(b)
  Subsystem4/7(Out7) -> Subtract36/2
  Subtract26/1 -> Product20/2, Product20/1
  Subsystem3/3(Out3) -> Subtract4/2
  Product28/1 -> Add5/1
  Product12/1 -> Add13/2
  Product8/1 -> Add16/1
  Product7/1 -> Add15/1
  Subsystem4/5(Out5) -> Subtract38/2
  Subsystem3/4(Out4) -> Subtract5/2
  Product21/1 -> Add7/2
  Subtract25/1 -> Product21/2, Product21/1
  Add6/1 -> Subsystem6/6(b2)
  Add13/1 -> Subsystem1/4(b1)
  Add2/1 -> Subsystem6/2(b)
  Product15/1 -> Add10/2
  Product14/1 -> Add11/2
  Add8/1 -> Subsystem6/8(b3)
  Product27/1 -> Add1/2
  Subsystem3/1(Out1) -> Subtract2/2
  Subtract42/1 -> Product8/1, Product8/2
  Subtract36/1 -> Product1/1, Product1/2
  Subtract23/1 -> Product23/1, Product23/2
  Add10/1 -> Subsystem1/7(a3)
  imag/1 -> Subtract42/1, Subtract39/1, Subtract28/1, Subtract36/1, Subtract37/1, Subtract38/1, Subtract40/1, Subtract41/1, Subtract9/1, Subtract8/1, Subtract7/1, Subtract6/1, Subtract5/1, Subtract4/1, Subtract3/1, Subtract2/1  "y"
  Add16/1 -> Subsystem1/1(a)
  Subtract2/1 -> Product32/2, Product32/1
  Subtract6/1 -> Product28/2, Product28/1
  Subtract5/1 -> Product29/1, Product29/2
  Product18/1 -> Add7/1
  Add9/1 -> Subsystem1/8(b3)
  Product30/1 -> Add3/1
  Subsystem3/5(Out5) -> Subtract6/2
  Product31/1 -> Add2/1
  Subtract19/1 -> Product27/2, Product27/1
  Product26/1 -> Add2/2
  Add11/1 -> Subsystem1/6(b2)
  Subsystem3/2(Out2) -> Subtract3/2
  Product22/1 -> Add6/2
  Subsystem1/1(min) -> Subtract18/2
  Product5/1 -> Add13/1
  Subtract18/1 -> Product2/1
  Subsystem4/6(Out6) -> Subtract37/2
  Subtract4/1 -> Product30/2, Product30/1
  Subtract24/1 -> Product22/2, Product22/1
  Add14/1 -> Subsystem1/3(a1)
  LLR Scale/1 -> Product2/2
  Product4/1 -> Add12/1
  Subtract21/1 -> Product25/2, Product25/1
  Product23/1 -> Add5/2
  Add7/1 -> Subsystem6/7(a3)
  Product3/1 -> Add11/1
  Product19/1 -> Add6/1
  Product25/1 -> Add3/2
  real/1 -> Subtract27/1, Subtract29/1, Subtract30/1, Subtract31/1, Subtract32/1, Subtract33/1, Subtract34/1, Subtract35/1, Subtract20/1, Subtract26/1, Subtract25/1, Subtract24/1, Subtract23/1, Subtract22/1, Subtract21/1, Subtract19/1  "X"
  Subtract35/1 -> Product9/1, Product9/2
  Subtract41/1 -> Product7/1, Product7/2
  Subsystem3/6(Out6) -> Subtract7/2
  Subsystem6/1(min) -> Subtract18/1
  Add3/1 -> Subsystem6/3(a1)
  Product20/1 -> Add8/2
  Add1/1 -> Subsystem6/1(a)
  Product/1 -> Add9/1
  Subtract38/1 -> Product4/2, Product4/1
  Product1/1 -> Add10/1
  Add12/1 -> Subsystem1/5(a2)
  Product10/1 -> Add15/2
  Product6/1 -> Add14/1
  Subsystem5/4(Out4) -> Subtract32/2

== system lib_rfsoc_fec/Soft Demodulation/sign_extend ==
  u : Inport
  Bit Concat : hdlsllib/Logic and Bit Operations/Bit Concat  numInputs=3
  Bit Slice : hdlsllib/Logic and Bit Operations/Bit Slice  lidx=5  ridx=5
      settings: SourceProductBaseCode=SL
  y : Outport
  wires:
  Bit Concat/1 -> y/1
  u/1 -> Bit Concat/3, Bit Slice/1
  Bit Slice/1 -> Bit Concat/2, Bit Concat/1

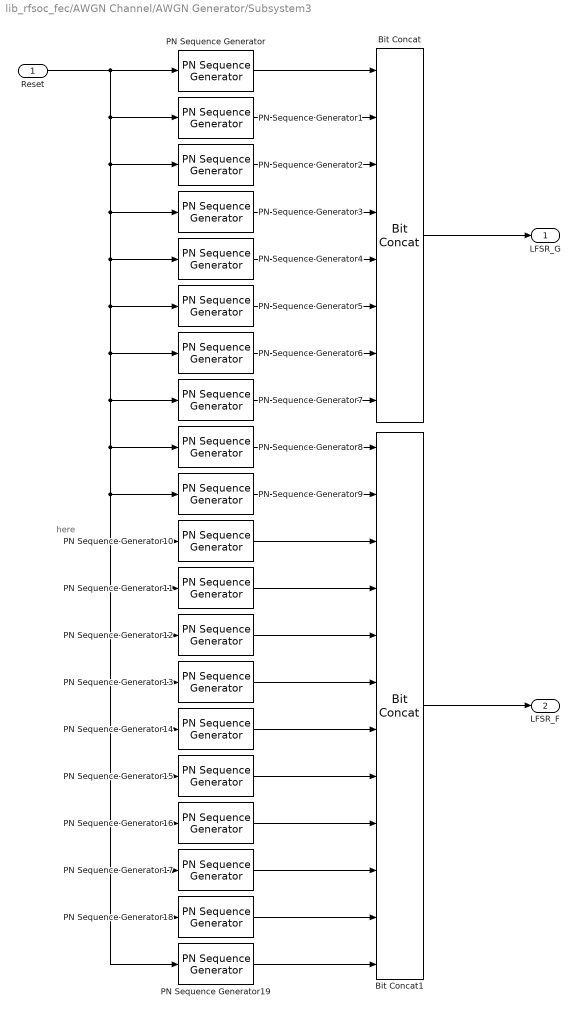
== system lib_rfsoc_fec/AWGN Channel/AWGN Generator/Subsystem3 ==
  note: here
  Reset : Inport
  Bit Concat : hdlsllib/Logic and Bit Operations/Bit Concat  numInputs=8
  Bit Concat1 : hdlsllib/Logic and Bit Operations/Bit Concat  numInputs=12
  PN Sequence Generator : commseqgen3/PN Sequence Generator  poly='z^13 + z^12 + z^11 + z^8 + 1'  ini_sta=[0 1 1 0 0 0 0 0 0 1 0 0 0]  outBitMaskSource=Dialog parameter  shift=0  outVarSiz=off  maxOutSizeMode=Dialog parameter  maxOutSize=[10 1]  Ts=-1  sampPerFrame=1  reset=on  bitPackedOutputs=off  outDataType=boolean  numPackedBits=8  bitPackDataSigned=off  bitPackedOutDType=Smallest integer
  PN Sequence Generator1 : commseqgen3/PN Sequence Generator  poly='z^13 + z^12 + z^11 + z^8 + 1'  ini_sta=[0 0 1 1 0 0 0 0 0 0 0 1 1]  outBitMaskSource=Dialog parameter  shift=0  outVarSiz=off  maxOutSizeMode=Dialog parameter  maxOutSize=[10 1]  Ts=-1  sampPerFrame=1  reset=on  bitPackedOutputs=off  outDataType=boolean  numPackedBits=8  bitPackDataSigned=off  bitPackedOutDType=Smallest integer
  PN Sequence Generator10 : commseqgen3/PN Sequence Generator  poly='z^13 + z^12 + z^11 + z^8 + 1'  ini_sta=[1 0 0 0 0 0 1 0 0 0 0 0 1]  outBitMaskSource=Dialog parameter  shift=0  outVarSiz=off  maxOutSizeMode=Dialog parameter  maxOutSize=[10 1]  Ts=-1  sampPerFrame=1  reset=on  bitPackedOutputs=off  outDataType=boolean  numPackedBits=8  bitPackDataSigned=off  bitPackedOutDType=Smallest integer
  PN Sequence Generator11 : commseqgen3/PN Sequence Generator  poly='z^13 + z^12 + z^11 + z^8 + 1'  ini_sta=[1 0 0 0 0 0 0 0 0 0 0 0 1]  outBitMaskSource=Dialog parameter  shift=0  outVarSiz=off  maxOutSizeMode=Dialog parameter  maxOutSize=[10 1]  Ts=-1  sampPerFrame=1  reset=on  bitPackedOutputs=off  outDataType=boolean  numPackedBits=8  bitPackDataSigned=off  bitPackedOutDType=Smallest integer
  PN Sequence Generator12 : commseqgen3/PN Sequence Generator  poly='z^13 + z^12 + z^11 + z^8 + 1'  ini_sta=[1 0 0 1 0 0 0 0 0 1 0 0 1]  outBitMaskSource=Dialog parameter  shift=0  outVarSiz=off  maxOutSizeMode=Dialog parameter  maxOutSize=[10 1]  Ts=-1  sampPerFrame=1  reset=on  bitPackedOutputs=off  outDataType=boolean  numPackedBits=8  bitPackDataSigned=off  bitPackedOutDType=Smallest integer
  PN Sequence Generator13 : commseqgen3/PN Sequence Generator  poly='z^13 + z^12 + z^11 + z^8 + 1'  ini_sta=[1 1 1 1 1 1 0 1 1 1 1 1 1]  outBitMaskSource=Dialog parameter  shift=0  outVarSiz=off  maxOutSizeMode=Dialog parameter  maxOutSize=[10 1]  Ts=-1  sampPerFrame=1  reset=on  bitPackedOutputs=off  outDataType=boolean  numPackedBits=8  bitPackDataSigned=off  bitPackedOutDType=Smallest integer
  PN Sequence Generator14 : commseqgen3/PN Sequence Generator  poly='z^13 + z^12 + z^11 + z^8 + 1'  ini_sta=[1 0 1 0 1 0 1 0 1 0 1 0 1]  outBitMaskSource=Dialog parameter  shift=0  outVarSiz=off  maxOutSizeMode=Dialog parameter  maxOutSize=[10 1]  Ts=-1  sampPerFrame=1  reset=on  bitPackedOutputs=off  outDataType=boolean  numPackedBits=8  bitPackDataSigned=off  bitPackedOutDType=Smallest integer
  PN Sequence Generator15 : commseqgen3/PN Sequence Generator  poly='z^13 + z^12 + z^11 + z^8 + 1'  ini_sta=[0 1 0 1 0 1 0 1 0 1 0 1 0]  outBitMaskSource=Dialog parameter  shift=0  outVarSiz=off  maxOutSizeMode=Dialog parameter  maxOutSize=[10 1]  Ts=-1  sampPerFrame=1  reset=on  bitPackedOutputs=off  outDataType=boolean  numPackedBits=8  bitPackDataSigned=off  bitPackedOutDType=Smallest integer
  PN Sequence Generator16 : commseqgen3/PN Sequence Generator  poly='z^13 + z^12 + z^11 + z^8 + 1'  ini_sta=[1 1 1 0 0 0 1 1 1 0 0 0 1]  outBitMaskSource=Dialog parameter  shift=0  outVarSiz=off  maxOutSizeMode=Dialog parameter  maxOutSize=[10 1]  Ts=-1  sampPerFrame=1  reset=on  bitPackedOutputs=off  outDataType=boolean  numPackedBits=8  bitPackDataSigned=off  bitPackedOutDType=Smallest integer
  PN Sequence Generator17 : commseqgen3/PN Sequence Generator  poly='z^13 + z^12 + z^11 + z^8 + 1'  ini_sta=[0 0 0 0 0 1 1 0 0 0 1 1 1]  outBitMaskSource=Dialog parameter  shift=0  outVarSiz=off  maxOutSizeMode=Dialog parameter  maxOutSize=[10 1]  Ts=-1  sampPerFrame=1  reset=on  bitPackedOutputs=off  outDataType=boolean  numPackedBits=8  bitPackDataSigned=off  bitPackedOutDType=Smallest integer
  PN Sequence Generator18 : commseqgen3/PN Sequence Generator  poly='z^13 + z^12 + z^11 + z^8 + 1'  ini_sta=[1 1 0 0 0 1 1 1 1 0 0 0 0]  outBitMaskSource=Dialog parameter  shift=0  outVarSiz=off  maxOutSizeMode=Dialog parameter  maxOutSize=[10 1]  Ts=-1  sampPerFrame=1  reset=on  bitPackedOutputs=off  outDataType=boolean  numPackedBits=8  bitPackDataSigned=off  bitPackedOutDType=Smallest integer
  PN Sequence Generator19 : commseqgen3/PN Sequence Generator  poly='z^13 + z^12 + z^11 + z^8 + 1'  ini_sta=[1 1 1 1 1 1 1 0 0 0 0 0 0]  outBitMaskSource=Dialog parameter  shift=0  outVarSiz=off  maxOutSizeMode=Dialog parameter  maxOutSize=[10 1]  Ts=-1  sampPerFrame=1  reset=on  bitPackedOutputs=off  outDataType=boolean  numPackedBits=8  bitPackDataSigned=off  bitPackedOutDType=Smallest integer
  PN Sequence Generator2 : commseqgen3/PN Sequence Generator  poly='z^13 + z^12 + z^11 + z^8 + 1'  ini_sta=[1 1 0 1 0 0 0 0 0 1 0 0 1]  outBitMaskSource=Dialog parameter  shift=0  outVarSiz=off  maxOutSizeMode=Dialog parameter  maxOutSize=[10 1]  Ts=-1  sampPerFrame=1  reset=on  bitPackedOutputs=off  outDataType=boolean  numPackedBits=8  bitPackDataSigned=off  bitPackedOutDType=Smallest integer
  PN Sequence Generator3 : commseqgen3/PN Sequence Generator  poly='z^13 + z^12 + z^11 + z^8 + 1'  ini_sta=[1 0 1 0 0 0 0 1 0 0 1 1 0]  outBitMaskSource=Dialog parameter  shift=0  outVarSiz=off  maxOutSizeMode=Dialog parameter  maxOutSize=[10 1]  Ts=-1  sampPerFrame=1  reset=on  bitPackedOutputs=off  outDataType=boolean  numPackedBits=8  bitPackDataSigned=off  bitPackedOutDType=Smallest integer
  PN Sequence Generator4 : commseqgen3/PN Sequence Generator  poly='z^13 + z^12 + z^11 + z^8 + 1'  ini_sta=[0 0 0 0 1 0 0 0 0 1 1 1 0]  outBitMaskSource=Dialog parameter  shift=0  outVarSiz=off  maxOutSizeMode=Dialog parameter  maxOutSize=[10 1]  Ts=-1  sampPerFrame=1  reset=on  bitPackedOutputs=off  outDataType=boolean  numPackedBits=8  bitPackDataSigned=off  bitPackedOutDType=Smallest integer
  PN Sequence Generator5 : commseqgen3/PN Sequence Generator  poly='z^13 + z^12 + z^11 + z^8 + 1'  ini_sta=[1 1 0 0 1 1 0 0 1 0 1 0 0]  outBitMaskSource=Dialog parameter  shift=0  outVarSiz=off  maxOutSizeMode=Dialog parameter  maxOutSize=[10 1]  Ts=-1  sampPerFrame=1  reset=on  bitPackedOutputs=off  outDataType=boolean  numPackedBits=8  bitPackDataSigned=off  bitPackedOutDType=Smallest integer
  PN Sequence Generator6 : commseqgen3/PN Sequence Generator  poly='z^13 + z^12 + z^11 + z^8 + 1'  ini_sta=[1 0 0 0 0 1 0 0 0 0 1 1 1]  outBitMaskSource=Dialog parameter  shift=0  outVarSiz=off  maxOutSizeMode=Dialog parameter  maxOutSize=[10 1]  Ts=-1  sampPerFrame=1  reset=on  bitPackedOutputs=off  outDataType=boolean  numPackedBits=8  bitPackDataSigned=off  bitPackedOutDType=Smallest integer
  PN Sequence Generator7 : commseqgen3/PN Sequence Generator  poly='z^13 + z^12 + z^11 + z^8 + 1'  ini_sta=[1 0 0 1 1 1 1 1 0 0 0 1 1]  outBitMaskSource=Dialog parameter  shift=0  outVarSiz=off  maxOutSizeMode=Dialog parameter  maxOutSize=[10 1]  Ts=-1  sampPerFrame=1  reset=on  bitPackedOutputs=off  outDataType=boolean  numPackedBits=8  bitPackDataSigned=off  bitPackedOutDType=Smallest integer
  PN Sequence Generator8 : commseqgen3/PN Sequence Generator  poly='z^13 + z^12 + z^11 + z^8 + 1'  ini_sta=[1 1 0 1 1 1 1 1 0 0 0 1 1]  outBitMaskSource=Dialog parameter  shift=0  outVarSiz=off  maxOutSizeMode=Dialog parameter  maxOutSize=[10 1]  Ts=-1  sampPerFrame=1  reset=on  bitPackedOutputs=off  outDataType=boolean  numPackedBits=8  bitPackDataSigned=off  bitPackedOutDType=Smallest integer
  PN Sequence Generator9 : commseqgen3/PN Sequence Generator  poly='z^13 + z^12 + z^11 + z^8 + 1'  ini_sta=[0 1 0 1 1 0 0 1 0 0 0 1 1]  outBitMaskSource=Dialog parameter  shift=0  outVarSiz=off  maxOutSizeMode=Dialog parameter  maxOutSize=[10 1]  Ts=-1  sampPerFrame=1  reset=on  bitPackedOutputs=off  outDataType=boolean  numPackedBits=8  bitPackDataSigned=off  bitPackedOutDType=Smallest integer
  LFSR_G : Outport
  LFSR_F : Outport  Port=2
  wires:
  PN Sequence Generator11/1 -> Bit Concat1/4
  PN Sequence Generator10/1 -> Bit Concat1/3
  PN Sequence Generator9/1 -> Bit Concat1/2
  PN Sequence Generator8/1 -> Bit Concat1/1
  Bit Concat1/1 -> LFSR_F/1
  Bit Concat/1 -> LFSR_G/1
  Reset/1 -> PN Sequence Generator/1, PN Sequence Generator2/1, PN Sequence Generator3/1, PN Sequence Generator8/1, PN Sequence Generator9/1, PN Sequence Generator11/1, PN Sequence Generator18/1, PN Sequence Generator19/1, PN Sequence Generator17/1, PN Sequence Generator16/1, PN Sequence Generator15/1, PN Sequence Generator14/1, PN Sequence Generator13/1, PN Sequence Generator12/1, PN Sequence Generator10/1, PN Sequence Generator7/1, PN Sequence Generator6/1, PN Sequence Generator5/1, PN Sequence Generator4/1, PN Sequence Generator1/1
  PN Sequence Generator18/1 -> Bit Concat1/11
  PN Sequence Generator13/1 -> Bit Concat1/6
  PN Sequence Generator14/1 -> Bit Concat1/7
  PN Sequence Generator12/1 -> Bit Concat1/5
  PN Sequence Generator15/1 -> Bit Concat1/8
  PN Sequence Generator16/1 -> Bit Concat1/9
  PN Sequence Generator17/1 -> Bit Concat1/10
  PN Sequence Generator19/1 -> Bit Concat1/12
  PN Sequence Generator7/1 -> Bit Concat/8
  PN Sequence Generator6/1 -> Bit Concat/7
  PN Sequence Generator5/1 -> Bit Concat/6
  PN Sequence Generator2/1 -> Bit Concat/3
  PN Sequence Generator1/1 -> Bit Concat/2
  PN Sequence Generator4/1 -> Bit Concat/5
  PN Sequence Generator3/1 -> Bit Concat/4
  PN Sequence Generator/1 -> Bit Concat/1

== system lib_rfsoc_fec/AWGN Channel/sample_and_hold/tvalid hold ==
  In1 : Inport
  Compare To Constant : simulink/Logic and Bit Operations/Compare To Constant  relop===  const=7  OutDataTypeStr=boolean
  Delay1 : Delay  DelayLength=1
  HDL Counter : hdlsllib/Sources/HDL Counter  CountType=Count limited  CountInit=0  CountStep=1  CountMax=7  CountFromType=Initial value  CountFrom=0  CountResetPort=off  CountLoadPort=off  CountEnbPort=on  CountDirPort=off  CountDataType=Unsigned  CountWordLen=3  CountFracLen=0  CountSampTime=1
  OR : Logic  Operator=OR  IconShape=distinctive  AllPortsSameDT=off  OutDataTypeStr=boolean
  Sample and Hold1 : dspsigops/Sample and Hold  trig=Rising edge  initCond=0  latchinput=off
  " " : Outport
  wires:
  HDL Counter/1 -> Compare To Constant/1
  Delay1/1 -> OR/1
  OR/1 -> Sample and Hold1/Trigger
  Compare To Constant/1 -> Delay1/1
  Sample and Hold1/1 -> " "/1, HDL Counter/1
  In1/1 -> Sample and Hold1/1, OR/2

== system lib_rfsoc_fec/QAM Mapping/sample_and_hold/tvalid hold ==
  In1 : Inport
  Compare To Constant : simulink/Logic and Bit Operations/Compare To Constant  relop===  const=7  OutDataTypeStr=boolean
  Delay1 : Delay  DelayLength=1
  HDL Counter : hdlsllib/Sources/HDL Counter  CountType=Count limited  CountInit=0  CountStep=1  CountMax=7  CountFromType=Initial value  CountFrom=0  CountResetPort=off  CountLoadPort=off  CountEnbPort=on  CountDirPort=off  CountDataType=Unsigned  CountWordLen=3  CountFracLen=0  CountSampTime=1
  OR : Logic  Operator=OR  IconShape=distinctive  AllPortsSameDT=off  OutDataTypeStr=boolean
  Sample and Hold1 : dspsigops/Sample and Hold  trig=Rising edge  initCond=0  latchinput=off
  " " : Outport
  wires:
  HDL Counter/1 -> Compare To Constant/1
  Delay1/1 -> OR/1
  OR/1 -> Sample and Hold1/Trigger
  Compare To Constant/1 -> Delay1/1
  Sample and Hold1/1 -> " "/1, HDL Counter/1
  In1/1 -> Sample and Hold1/1, OR/2

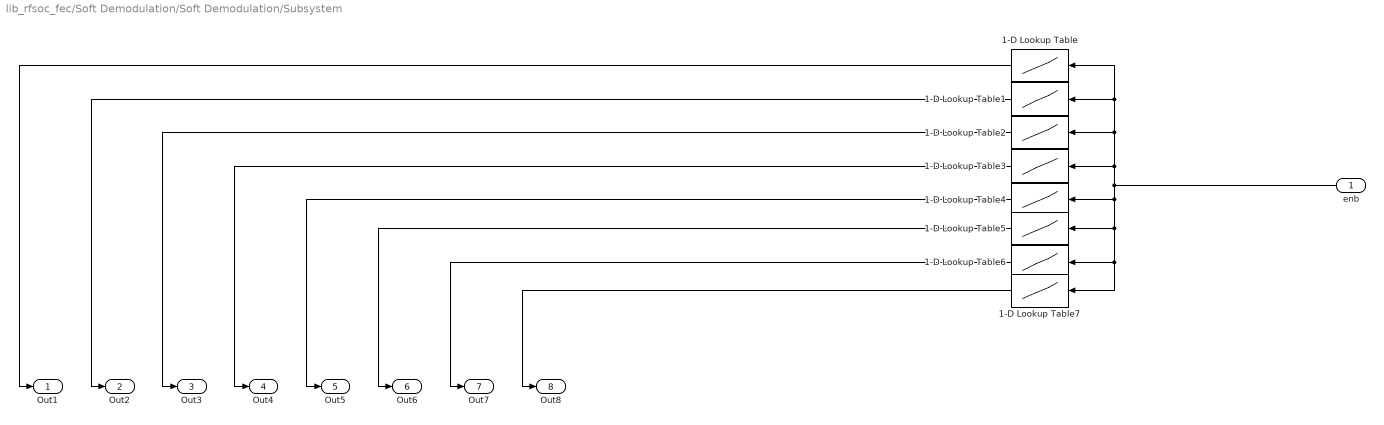
== system lib_rfsoc_fec/Soft Demodulation/Soft Demodulation/Subsystem ==
  enb : Inport
  1-D Lookup Table : Lookup_n-D  NumberOfTableDimensions=1  BreakpointsForDimension1=[0:3]  IndexSearchMethod=Evenly spaced points  Table=[3 3 3 -1]  InterpMethod=Flat  DiagnosticForOutOfRangeInput=Error  InternalRulePriority=Speed  OutDataTypeStr=fixdt(1,3,0)  RndMeth=Simplest  InputSameDT=on
  1-D Lookup Table1 : Lookup_n-D  NumberOfTableDimensions=1  BreakpointsForDimension1=[0:3]  IndexSearchMethod=Evenly spaced points  Table=[1 1 3 -1]  InterpMethod=Flat  DiagnosticForOutOfRangeInput=Error  InternalRulePriority=Speed  OutDataTypeStr=fixdt(1,3,0)  RndMeth=Simplest  InputSameDT=on
  1-D Lookup Table2 : Lookup_n-D  NumberOfTableDimensions=1  BreakpointsForDimension1=[0:3]  IndexSearchMethod=Evenly spaced points  Table=[-1 -1 3 -1]  InterpMethod=Flat  DiagnosticForOutOfRangeInput=Error  InternalRulePriority=Speed  OutDataTypeStr=fixdt(1,3,0)  RndMeth=Simplest  InputSameDT=on
  1-D Lookup Table3 : Lookup_n-D  NumberOfTableDimensions=1  BreakpointsForDimension1=[0:3]  IndexSearchMethod=Evenly spaced points  Table=[-3 -3 3 -1]  InterpMethod=Flat  DiagnosticForOutOfRangeInput=Error  InternalRulePriority=Speed  OutDataTypeStr=fixdt(1,3,0)  RndMeth=Simplest  InputSameDT=on
  1-D Lookup Table4 : Lookup_n-D  NumberOfTableDimensions=1  BreakpointsForDimension1=[0:3]  IndexSearchMethod=Evenly spaced points  Table=[3 3 -3 -3]  InterpMethod=Flat  DiagnosticForOutOfRangeInput=Error  InternalRulePriority=Speed  OutDataTypeStr=fixdt(1,3,0)  RndMeth=Simplest  InputSameDT=on
  1-D Lookup Table5 : Lookup_n-D  NumberOfTableDimensions=1  BreakpointsForDimension1=[0:3]  IndexSearchMethod=Evenly spaced points  Table=[1 1 -3 -3]  InterpMethod=Flat  DiagnosticForOutOfRangeInput=Error  InternalRulePriority=Speed  OutDataTypeStr=fixdt(1,3,0)  RndMeth=Simplest  InputSameDT=on
  1-D Lookup Table6 : Lookup_n-D  NumberOfTableDimensions=1  BreakpointsForDimension1=[0:3]  IndexSearchMethod=Evenly spaced points  Table=[-1 -1 -3 -3]  InterpMethod=Flat  DiagnosticForOutOfRangeInput=Error  InternalRulePriority=Speed  OutDataTypeStr=fixdt(1,3,0)  RndMeth=Simplest  InputSameDT=on
  1-D Lookup Table7 : Lookup_n-D  NumberOfTableDimensions=1  BreakpointsForDimension1=[0:3]  IndexSearchMethod=Evenly spaced points  Table=[-3 -3 -3 -3]  InterpMethod=Flat  DiagnosticForOutOfRangeInput=Error  InternalRulePriority=Speed  OutDataTypeStr=fixdt(1,3,0)  RndMeth=Simplest  InputSameDT=on
  Out1 : Outport
  Out2 : Outport  Port=2
  Out3 : Outport  Port=3
  Out4 : Outport  Port=4
  Out5 : Outport  Port=5
  Out6 : Outport  Port=6
  Out7 : Outport  Port=7
  Out8 : Outport  Port=8
  wires:
  1-D Lookup Table7/1 -> Out8/1
  1-D Lookup Table2/1 -> Out3/1
  1-D Lookup Table/1 -> Out1/1
  1-D Lookup Table5/1 -> Out6/1
  1-D Lookup Table4/1 -> Out5/1
  1-D Lookup Table1/1 -> Out2/1
  1-D Lookup Table3/1 -> Out4/1
  enb/1 -> 1-D Lookup Table7/1, 1-D Lookup Table6/1, 1-D Lookup Table5/1, 1-D Lookup Table4/1, 1-D Lookup Table/1, 1-D Lookup Table1/1, 1-D Lookup Table2/1, 1-D Lookup Table3/1
  1-D Lookup Table6/1 -> Out7/1

== system lib_rfsoc_fec/Soft Demodulation/Soft Demodulation/Subsystem1 ==
  a : Inport
  b : Inport  Port=2
  a1 : Inport  Port=3
  b1 : Inport  Port=4
  a2 : Inport  Port=5
  b2 : Inport  Port=6
  a3 : Inport  Port=7
  b3 : Inport  Port=8
  get_min1 : Subsystem
  get_min2 : Subsystem
  get_min3 : Subsystem
  get_min4 : Subsystem
  get_min5 : Subsystem
  get_min6 : Subsystem
  get_min7 : Subsystem
  min : Outport
  wires:
  a2/1 -> get_min3/1(a)
  b/1 -> get_min1/2(b)
  a1/1 -> get_min2/1(a)
  b3/1 -> get_min4/2(b)
  get_min7/1(min) -> min/1
  get_min1/1(min) -> get_min5/1(a)
  a3/1 -> get_min4/1(a)
  get_min4/1(min) -> get_min6/2(b)
  get_min2/1(min) -> get_min5/2(b)
  b1/1 -> get_min2/2(b)
  get_min3/1(min) -> get_min6/1(a)
  get_min6/1(min) -> get_min7/2(b)
  a/1 -> get_min1/1(a)
  b2/1 -> get_min3/2(b)
  get_min5/1(min) -> get_min7/1(a)
